simulink model "gm_flanger_short"  (R2018a)
settings: Solver=FixedStepDiscrete  StartTime=0.0  StopTime=10.0  RelTol=1e-3
libraries: dspvision x2, dspsigops x1
settings Model: Creator=Lu  LastModifiedBy=Lu
settings DataIOCC: SaveOutput=off  SaveTime=off
settings OptimizationCC: BlockReduction=off  ConditionallyExecuteInputs=off  DefaultParameterBehavior=Inlined
settings DebuggingCC: AlgebraicLoopMsg=error  SingleTaskRateTransMsg=error
settings HardwareCC: ProdBitPerPointer=32  ProdBitPerSizeT=32  ProdBitPerPtrDiffT=32  ProdLargestAtomicFloat=None  ProdIntDivRoundTo=Undefined  ProdEndianess=Unspecified  ProdWordSize=32  ProdHWDeviceType=ASIC/FPGA->ASIC/FPGA  TargetBitPerPointer=64  TargetBitPerSizeT=64  TargetBitPerPtrDiffT=64  TargetLongLongMode=on  TargetIntDivRoundTo=Zero  TargetEndianess=LittleEndian  TargetWordSize=64  TargetHWDeviceType=Custom Processor->MATLAB Host Computer  ProdEqTarget=off

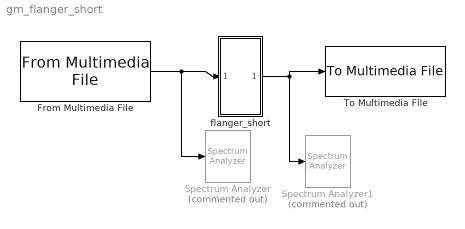
== system gm_flanger_short ==
  From Multimedia File : dspvision/From Multimedia File  inputFilename=C:\Users\lugfe\Documents\GitHub\dsp-fpgay\TP FINAL\audio effects\shook.wav  loop=on  numPlays=1  outputStreams=Audio only  videoDataType=single  audioDataType=int16  inheritSampleTime=on  userDefinedSampleTime=1/30  noAudioOutput=off  isIntensityVideo=off  fourcc=RGB  colorVideoFormat=Separate color signals  outputEOF=off  dataOrg=Column-major  audioFrameSize=1  computeAudioFrameSize=off  outSamplingMode=Sample based
      settings: SourceProductBaseCode=VP
  Spectrum Analyzer : SpectrumAnalyzer  Commented=on
  Spectrum Analyzer1 : SpectrumAnalyzer  Commented=on
  To Multimedia File : dspvision/To Multimedia File  outputFilename=C:\Users\lugfe\Documents\GitHub\dsp-fpgay\TP FINAL\audio effects\flanger_shook.wav  streamSelection=Audio only  videoCompressor=None (uncompressed)  audioCompressor=None (uncompressed)  imagePorts=Separate color signals  fileType=WAV  audioDatatype=Determine from input data type  fourcc=RGB  videoQuality=75  mj2000CompFactor=10
      settings: SourceProductName=Computer Vision System Toolbox  SourceProductBaseCode=VP
  "flanger_short " : Subsystem
  wires:
  From Multimedia File/1 -> Spectrum Analyzer/1, "flanger_short "/1(In2)
  "flanger_short "/1(Out2) -> To Multimedia File/1, Spectrum Analyzer1/1

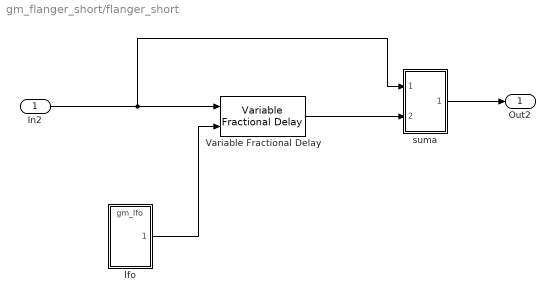
== system gm_flanger_short/flanger_short  ==
  In2 : Inport  OutDataTypeStr=int16  SampleTime=1/44100
  Variable Fractional Delay : dspsigops/Variable Fractional Delay  mode=OBSOLETE  modeActive=Linear  dmax=2000  InputProcessing=Columns as channels (frame based)  L=4  FarrowL=4  R=10  alpha=1  ic=0  fallbackFIR=Clip to the minimum value necessary for centered kernel  fallbackFarrow=Clip to the minimum value necessary for centered kernel  noDFT=off  roundingMode=Ceiling  overflowMode=on
      settings: SourceProductName=DSP System Toolbox  SourceProductBaseCode=DS
  lfo : ModelReference  ModelNameDialog=gm_lfo  SimulationMode=Normal  Variant=on  OverrideUsingVariant=HDLC_internal_variant_GeneratedDUT  ModelReferenceVersion=1.113
  "suma " : Subsystem
  Out2 : Outport
  wires:
  In2/1 -> "suma "/1(In1), Variable Fractional Delay/1
  "suma "/1(Out1) -> Out2/1
  Variable Fractional Delay/1 -> "suma "/2(In2)
  lfo/1 -> Variable Fractional Delay/2

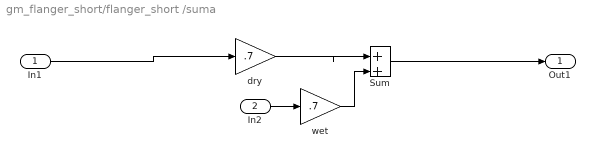
== system gm_flanger_short/flanger_short /suma  ==
  In1 : Inport
  In2 : Inport  Port=2
  Sum : Sum  Inputs=|++  AccumDataTypeStr=int16
  dry : Gain  Gain=.7  OutDataTypeStr=int16
  wet : Gain  Gain=.7  OutDataTypeStr=int16
  Out1 : Outport
  wires:
  In2/1 -> wet/1
  Sum/1 -> Out1/1
  In1/1 -> dry/1
  wet/1 -> Sum/2
  dry/1 -> Sum/1
